simulink model "lift_5_floor"  (R2020a)
settings: Solver=VariableStepAuto  StartTime=0.0  StopTime=10.0  RelTol=1e-3
settings Model: Creator=Shubham  LastModifiedBy=Shubham

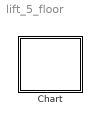
== system lift_5_floor ==
  Chart : Stateflow chart  TreatAsAtomicUnit=on

== stateflow chart lift_5_floor/Chart ==
  state first_floor
    f=1;
  state second_floor
    f=2;
  state Ground_floor
    f=0;
  state third_floor
    f=3;
  state fifth_floor
    f=5;
  state fourth_floor
    f=4;
  second_floor -> third_floor [order 2] : {f=3}
  first_floor -> second_floor [order 1] : {f=2}
  Ground_floor -> first_floor : {f=1}
  third_floor -> second_floor [order 1] : {f=2}
  second_floor -> first_floor [order 1] : {f=1}
  first_floor -> Ground_floor [order 2] : {f=0}
  (default) -> Ground_floor
  third_floor -> fourth_floor [order 2] : {f=4}
  fourth_floor -> third_floor [order 1] : {f=3}
  fifth_floor -> fourth_floor : {f=4}
  fourth_floor -> fifth_floor [order 2] : {f=5}
